simulink model "rpi_long_ctrl"  (R2022b)
settings: Solver=FixedStepAuto  StartTime=0.0  StopTime=15  RelTol=1e-3  EnableMultiTasking=on
values from neighbouring files (symbols this model uses):
  A = [1.06559801427  0.0478097134081  -0.0142426631232; 0.0478097134081  0.959164863261  -0.0359507847494; -0.0142426631232  -0.0359507847494  0.982079248423]    [matlab.mat]
  b = [2.14306210308 15.720848335 -0.863601368467]    [matlab.mat]
  D = 0    [matlab.mat]
  error_min = 0.04    [matlab.mat]
  I = 0    [matlab.mat]
  left_side = 0    [matlab.mat]
  N = 2    [matlab.mat]
  P = 1.25    [matlab.mat]
  pwm_k = 0.02    [matlab.mat]
  pwm_min = 0.27    [matlab.mat]
  pwm_min_ref = 0.25    [matlab.mat]
  target_scale = 0.75    [matlab.mat]
undefined symbols (not defined in the file or in its folder): ODR
libraries: raspberrypiBasiclib x6, simulink x2, raspberrypiIMUsensorslib x2, slpidlib x1, dspstat3 x1, dspsigops x1
settings Model: Creator=sjohnson  LastModifiedBy=sjohnson
settings SolverCC: PositivePriorityOrder=on
settings OptimizationCC: EnhancedBackFolding=on  PassReuseOutputArgsAs=Individual arguments  ZeroExternalMemoryAtStartup=off  ZeroInternalMemoryAtStartup=off  MaxStackSize=64  OptimizeBlockOrder=speed  DifferentSizesBufferReuse=on  OptimizationCustomize=off  EfficientTunableParamExpr=on
settings DebuggingCC: ParameterTunabilityLossMsg=error
settings HardwareCC: ProdBitPerPointer=32  ProdBitPerSizeT=32  ProdBitPerPtrDiffT=32  ProdLargestAtomicInteger=Long  ProdLargestAtomicFloat=Double  ProdWordSize=32  ProdLongLongMode=on  ProdHWDeviceType=ARM Compatible->ARM Cortex  UseEmbeddedCoderFeatures=off  UseSimulinkCoderFeatures=off
settings RTWCC: Description=Embedded Coder  SystemTargetFile=ert.tlc  HardwareBoard=Raspberry Pi  TLCOptions="-aInlineSetEventsForThisBaseRateFcn=TLC_FALSE -aSuppressMultiTaskScheduler=TLC_FALSE  -aRateBasedStepFcn=0"  TemplateMakefile=ert_default_tmf  Toolchain=GNU GCC Embedded Linux  BuildConfiguration=Faster Runs
settings CodeAppCC: ForceParamTrailComments=on  IgnoreCustomStorageClasses=off  OperatorAnnotations=on  SimulinkDataObjDesc=on  SFDataObjDesc=on  InsertBlockDesc=on
settings ERTTargetCC: SupportNonInlinedSFcns=on  SupportVariableSizeSignals=on  ExtModeTransport=2  ExtModeStaticAlloc=on  ExtModeMexFile=ext_xcp  ExtModeIntrfLevel=Level2 - Open

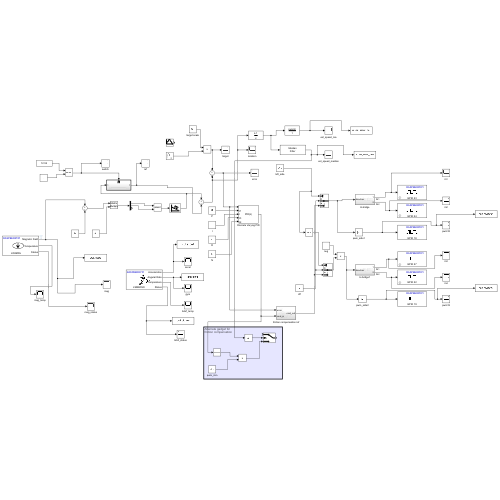
[thumbnail: Simulink's stored preview of the top-level diagram]
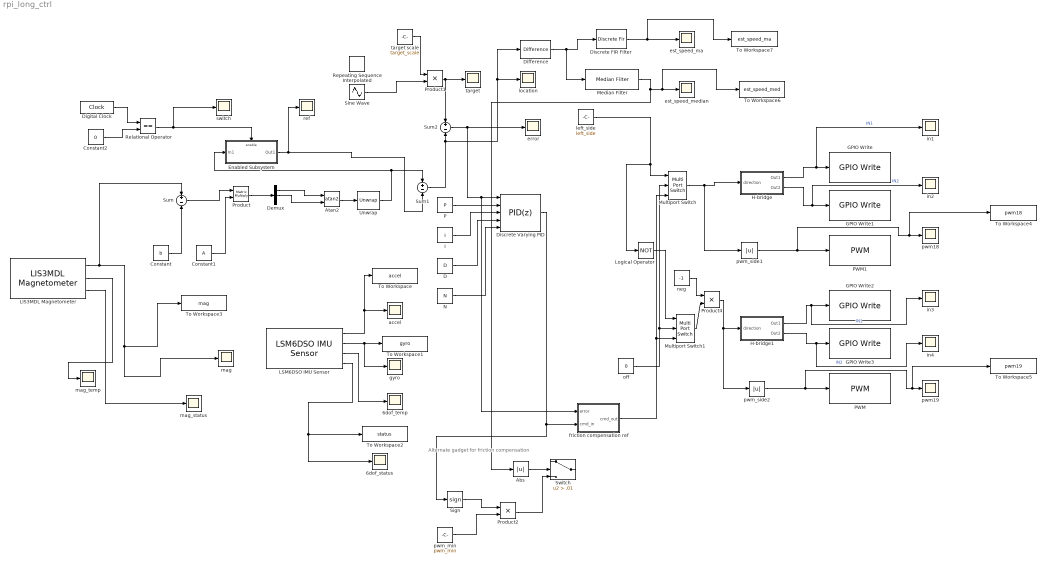
== system rpi_long_ctrl ==
  note: Alternate gadget for
      | friction compensation
  6dof_status : Scope
  6dof_temp : Scope
  Abs : Abs  SaturateOnIntegerOverflow=off
  Atan2 : Trigonometry  Operator=atan2
  Constant : Constant  Value=b
  Constant1 : Constant  Value=A
  Constant2 : Constant  Value=0
  D : Constant  Value=D
  Demux : Demux  Outputs=3
  Difference : simulink/Discrete/Difference  ICPrevInput=0  OutMin=[]  OutMax=[]  OutDataType=fixdt(1, 16)  OutScaling=2^-10  DoSatur=off
  Digital Clock : DigitalClock  SampleTime=0.04
  Discrete FIR Filter : DiscreteFir  Coefficients=[1 1 1 1 1]/5
  Discrete Varying PID : slpidlib/PID Controller  Controller=PID  Form=Parallel  TimeDomain=Discrete-time  UseExternalTs=off  SampleTime=-1  IntegratorMethod=Forward Euler  FilterMethod=Forward Euler  ControllerParametersSource=external  P=1  I=1  UseKiTs=off  D=0  N=100  UseFilter=on  TunerSelectOption=Transfer Function Based (PID Tuner App)  InitialConditionSource=internal  InitialConditionForIntegrator=0  InitialConditionForFilter=0  DifferentiatorICPrevScaledInput=0  ExternalReset=none  TrackingMode=off  Kt=1  LimitOutput=off  SatLimitsSource=internal  UpperSaturationLimit=inf  LowerSaturationLimit=-inf  LinearizeAsGain=on  AntiWindupMode=none  Kb=1  LimitIntegrator=off  UpperIntegratorSaturationLimit=inf  LowerIntegratorSaturationLimit=-inf  POutMin=[]  POutMax=[]  IOutMin=[]  IOutMax=[]  DOutMin=[]  DOutMax=[]  NOutMin=[]  NOutMax=[]  SumOutMin=[]  SumOutMax=[]  SaturationOutMin=[]  SaturationOutMax=[]  PParamMin=[]  PParamMax=[]  IParamMin=[]  IParamMax=[]  DParamMin=[]  DParamMax=[]  NParamMin=[]  NParamMax=[]  KbParamMin=[]  KbParamMax=[]  KtParamMin=[]  KtParamMax=[]  KbOutMin=[]  KbOutMax=[]  KtOutMin=[]  KtOutMax=[]  IntegratorOutMin=[]  IntegratorOutMax=[]  FilterOutMin=[]  FilterOutMax=[]  SumI1OutMin=[]  SumI1OutMax=[]  SumI2OutMin=[]  SumI2OutMax=[]  SumI3OutMin=[]  SumI3OutMax=[]  SumI4OutMin=[]  SumI4OutMax=[]  SumDOutMin=[]  SumDOutMax=[]  DifferentiatorOutMin=[]  DifferentiatorOutMax=[]  FilterDiffOutCoefMin=[]  FilterDiffOutCoefMax=[]  ReciprocalOutMin=[]  ReciprocalOutMax=[]  SumDenOutMin=[]  SumDenOutMax=[]  SumNumOutMin=[]  SumNumOutMax=[]  DivideOutMin=[]  DivideOutMax=[]  UdiffTsProdOutMin=[]  UdiffTsProdOutMax=[]  NTsProdOutMin=[]  NTsProdOutMax=[]  UintegralTsProdOutMin=[]  UintegralTsProdOutMax=[]  UngainTsProdOutMin=[]  UngainTsProdOutMax=[]  ClampingZeroOutDataTypeStr=Inherit: Inherit via back propagation  ClampingZeroOutMin=[]  ClampingZeroOutMax=[]  FilterDenConstantOutDataTypeStr=Inherit: Inherit via back propagation  FilterDenConstantOutMin=[]  FilterDenConstantOutMax=[]  PCopyOutDataTypeStr=Inherit: Inherit via back propagation  PCopyOutMin=[]  PCopyOutMax=[]  NCopyOutDataTypeStr=Inherit: Inherit via back propagation  NCopyOutMin=[]  NCopyOutMax=[]  IntegratorContinuousStateAttributes=''  IntegratorStateMustResolveToSignalObject=off  IntegratorRTWStateStorageClass=Auto  FilterContinuousStateAttributes=''  FilterStateMustResolveToSignalObject=off  FilterRTWStateStorageClass=Auto  ParallelPVariant=ExternalParameters  IdealPVariant=Disabled  IVariant=ExternalParameters  DVariant=ExternalParameters  IntegratorVariant=Discrete  SatVariant=Disabled  AWVariant=Passthrough  PCopyVariant=Disabled  TRVariant=Disabled  FdbkBlocksVariant=Forward  IdealPFdbkVariant=Disabled  SatFdbkVariant=Disabled  DerivativeFilterVariant=ForwardEulerFilter  NVariant=ExternalParameters  NCopyVariant=Disabled  FilterICVariant=InternalICsFilter  IntegratorICVariant=InternalICs  ExternalResetVariant=Disabled  TRSumVariant=Passthrough  SumFdbkVariant=Disabled  SumVariant=Sum_PID  TsampFilterVariant=InternalTs  TsampNgainVariant=Passthrough  TsampIntegralVariant=Passthrough  ExternalSaturationOutDataTypeStr=Inherit: Same as second input
      settings: LibrarySourceBlock=cstblocks/Linear Parameter Varying/Discrete Varying PID
  Enabled Subsystem : Subsystem  TreatAsAtomicUnit=on
  GPIO Write : raspberrypiBasiclib/GPIO Write  board=Pi 4 Model B  gpio=23  direction=Output  blockPlatform=Raspberry Pi
  GPIO Write1 : raspberrypiBasiclib/GPIO Write  board=Pi 4 Model B  gpio=24  direction=Output  blockPlatform=Raspberry Pi
  GPIO Write2 : raspberrypiBasiclib/GPIO Write  board=Pi 4 Model B  gpio=27  direction=Output  blockPlatform=Raspberry Pi
  GPIO Write3 : raspberrypiBasiclib/GPIO Write  board=Pi 4 Model B  gpio=22  direction=Output  blockPlatform=Raspberry Pi
  H-bridge : Subsystem
  H-bridge1 : Subsystem
  I : Constant  Value=I
  LIS3MDL Magnetometer : raspberrypiIMUsensorslib/LIS3MDL Magnetometer  I2CModule=1  I2CAddress=0x1E  IsActiveMagnetometer=on  IsActiveTemperature=on  IsStatus=on  SampleTime=-1  MagnetometerRange=+/- 400 uT  MagnetometerODR=40 Hz
  LSM6DSO IMU Sensor : raspberrypiIMUsensorslib/LSM6DSO IMU Sensor  I2CModule=1  I2CAddress=0x6B  IsActiveAcceleration=on  IsActiveAngularRate=on  IsActiveTemperature=on  IsActiveStatus=on  IsActiveTimeStamp=off  SampleTime=-1  QueueSizeFactor=3  AccelerometerRange=+/- 2g  AccelerometerODR=52 Hz  AccelSelectCompositeFilter=No filter  AccelLPF2BW=ODR/4  AccelHPFBW=ODR/4  GyroscopeRange=125 dps  GyroscopeODR=104 Hz  EnableGyroHPF=off  GyroHPFBW=0.016 Hz  EnableGyroLPF=off  GyroLPFBWMode=0
  Logical Operator : Logic  Operator=NOT  Inputs=1  AllPortsSameDT=off  OutDataTypeStr=boolean
  Median Filter : dspstat3/Median Filter  WindowLength=5  SimulateUsing=Interpreted execution
      settings: LibrarySourceBlock=|
      | dspfdesign/Median
      | Filter
  Multiport Switch : MultiPortSwitch  DataPortOrder=Zero-based contiguous  Inputs=2  zeroidx=on  SaturateOnIntegerOverflow=off  InputSameDT=off
  Multiport Switch1 : MultiPortSwitch  DataPortOrder=Zero-based contiguous  Inputs=2  zeroidx=on  SaturateOnIntegerOverflow=off  InputSameDT=off
  N : Constant  Value=N
  P : Constant  Value=P
  PWM : raspberrypiBasiclib/PWM  board=Pi 4 Model B  Pin_=19  Frequency=50  blockPlatform=Raspberry Pi
  PWM1 : raspberrypiBasiclib/PWM  board=Pi 4 Model B  Pin_=18  Frequency=50  blockPlatform=Raspberry Pi
  Product : Product  Multiplication=Matrix(*)
  Product1 : Product
  Product2 : Product
  Product4 : Product
  Relational Operator : RelationalOperator  Operator===  OutDataTypeStr=boolean  RndMeth=Simplest  InputSameDT=off
  Repeating Sequence Interpolated : simulink/Sources/Repeating Sequence Interpolated  OutValues=[0 pi/2 pi/2 pi pi pi/2 pi/2 0 0]  TimeValues=[0 1 2 3 4 5 6 7 8].'  LookUpMeth=Interpolation-Use End Values  tsamp=0.01  OutMin=[]  OutMax=[]  OutDataTypeStr=double  OutputDataTypeScalingMode=double  OutDataType=fixdt(0,8)  OutScaling=2^-10
  Sign : Signum
  Sine Wave : Sin  Amplitude=2*pi  Frequency=0.4  SampleTime=0.04
  Sum : Sum  Inputs=+-
  Sum1 : Sum  Inputs=+-
  Sum2 : Sum  Inputs=+-
  Switch : Switch  Criteria=u2 > Threshold  Threshold=.01  SaturateOnIntegerOverflow=off  InputSameDT=off
  To Workspace : ToWorkspace  VariableName=accel  SaveFormat=Structure With Time  SampleTime=-1
  To Workspace1 : ToWorkspace  VariableName=gyro  SaveFormat=Structure With Time  SampleTime=-1
  To Workspace2 : ToWorkspace  VariableName=status  SaveFormat=Structure With Time  SampleTime=-1
  To Workspace3 : ToWorkspace  VariableName=mag  SaveFormat=Structure With Time  SampleTime=-1
  To Workspace4 : ToWorkspace  VariableName=pwm18  SaveFormat=Structure With Time  SampleTime=-1
  To Workspace5 : ToWorkspace  VariableName=pwm19  SaveFormat=Structure With Time  SampleTime=-1
  To Workspace6 : ToWorkspace  VariableName=est_speed_med  SaveFormat=Structure With Time  SampleTime=-1
  To Workspace7 : ToWorkspace  VariableName=est_speed_ma  SaveFormat=Structure With Time  SampleTime=-1
  Unwrap : dspsigops/Unwrap  tol=pi  InputProcessing=Columns as channels (frame based)  running=off
  accel : Scope
  error : Scope
  est_speed_ma : Scope
  est_speed_median : Scope
  friction compensation ref : Subsystem
  gyro : Scope
  in{1..4} (4 alike) : Scope
  left_side : Constant  Value=left_side
  location : Scope
  mag : Scope
  mag_status : Scope
  mag_temp : Scope
  neg : Constant  Value=-1
  off : Constant  Value=0
  pwm18 : Scope
  pwm19 : Scope
  pwm_min : Constant  Value=pwm_min
  pwm_side1 : Abs  SaturateOnIntegerOverflow=off
  pwm_side2 : Abs  SaturateOnIntegerOverflow=off
  ref : Scope
  switch : Scope
  target : Scope
  target scale : Constant  Value=target_scale
  wires:
  Sine Wave/1 -> Product1/2
  LSM6DSO IMU Sensor/3 -> 6dof_temp/1
  LIS3MDL Magnetometer/3 -> mag_status/1
  LSM6DSO IMU Sensor/4 -> 6dof_status/1, To Workspace2/1
  LIS3MDL Magnetometer/1 -> Sum/1, To Workspace3/1, mag/1
  LSM6DSO IMU Sensor/1 -> accel/1, To Workspace/1
  LIS3MDL Magnetometer/2 -> mag_temp/1
  LSM6DSO IMU Sensor/2 -> gyro/1, To Workspace1/1
  Constant/1 -> Sum/2
  Sum/1 -> Product/1
  Constant1/1 -> Product/2
  Product/1 -> Demux/1
  Demux/1 -> Atan2/1
  Demux/2 -> Atan2/2
  Atan2/1 -> Unwrap/1
  Relational Operator/1 -> Enabled Subsystem/Enable, switch/1
  Digital Clock/1 -> Relational Operator/1
  Constant2/1 -> Relational Operator/2
  Enabled Subsystem/1(Out1) -> Sum1/2, ref/1
  Unwrap/1 -> Enabled Subsystem/1(In1), Sum1/1
  target scale/1 -> Product1/1
  Product1/1 -> target/1, Sum2/1
  off/1 -> Multiport Switch/2, Multiport Switch1/2
  Logical Operator/1 -> Multiport Switch1/1
  H-bridge1/2(Out2) -> in4/1, GPIO Write3/1  "IN2"
  left_side/1 -> Logical Operator/1, Multiport Switch/1
  pwm_side1/1 -> To Workspace4/1, pwm18/1, PWM1/1
  Product4/1 -> pwm_side2/1, H-bridge1/1(direction)
  pwm_side2/1 -> PWM/1, To Workspace5/1, pwm19/1
  H-bridge1/1(Out1) -> in3/1, GPIO Write2/1  "IN1"
  H-bridge/1(Out1) -> in1/1, GPIO Write/1  "IN1"
  Multiport Switch/1 -> pwm_side1/1, H-bridge/1(direction)
  H-bridge/2(Out2) -> in2/1, GPIO Write1/1  "IN2"
  Sum2/1 -> error/1, friction compensation ref/1(error), Discrete Varying PID/1
  P/1 -> Discrete Varying PID/2
  I/1 -> Discrete Varying PID/3
  D/1 -> Discrete Varying PID/4
  N/1 -> Discrete Varying PID/5
  neg/1 -> Product4/1
  Multiport Switch1/1 -> Product4/2
  Discrete Varying PID/1 -> Sign/1, friction compensation ref/2(cmd_in)
  Sum1/1 -> Difference/1, location/1, Sum2/2
  Difference/1 -> Median Filter/1, Discrete FIR Filter/1
  Discrete FIR Filter/1 -> To Workspace7/1, est_speed_ma/1
  Median Filter/1 -> Abs/1, To Workspace6/1, est_speed_median/1
  Abs/1 -> Switch/2
  Sign/1 -> Product2/1
  pwm_min/1 -> Product2/2
  Product2/1 -> Switch/3
  friction compensation ref/1(cmd_out) -> Multiport Switch1/3, Multiport Switch/3

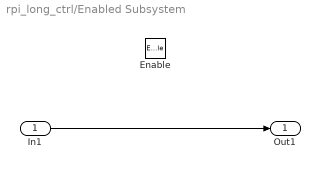
== system rpi_long_ctrl/Enabled Subsystem ==
  In1 : Inport
  Enable : EnablePort
  Out1 : Outport
  wires:
  In1/1 -> Out1/1

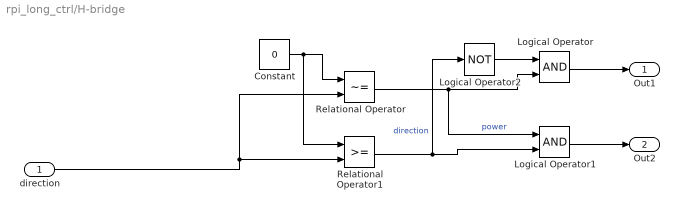
== system rpi_long_ctrl/H-bridge ==
  direction : Inport
  Constant : Constant  Value=0
  Logical Operator : Logic  AllPortsSameDT=off  OutDataTypeStr=boolean
  Logical Operator1 : Logic  AllPortsSameDT=off  OutDataTypeStr=boolean
  Logical Operator2 : Logic  Operator=NOT  Inputs=1  AllPortsSameDT=off  OutDataTypeStr=boolean
  Relational Operator : RelationalOperator  Operator=~=  OutDataTypeStr=boolean  RndMeth=Simplest  InputSameDT=off
  Relational Operator1 : RelationalOperator  OutDataTypeStr=boolean  RndMeth=Simplest  InputSameDT=off
  Out1 : Outport
  Out2 : Outport  Port=2
  wires:
  Logical Operator/1 -> Out1/1
  Relational Operator1/1 -> Logical Operator2/1, Logical Operator1/2  "direction"
  Logical Operator1/1 -> Out2/1
  Logical Operator2/1 -> Logical Operator/1
  direction/1 -> Relational Operator/2, Relational Operator1/2
  Constant/1 -> Relational Operator1/1, Relational Operator/1
  Relational Operator/1 -> Logical Operator1/1, Logical Operator/2  "power"

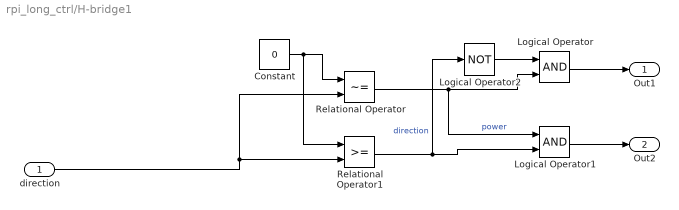
== system rpi_long_ctrl/H-bridge1 ==
  direction : Inport
  Constant : Constant  Value=0
  Logical Operator : Logic  AllPortsSameDT=off  OutDataTypeStr=boolean
  Logical Operator1 : Logic  AllPortsSameDT=off  OutDataTypeStr=boolean
  Logical Operator2 : Logic  Operator=NOT  Inputs=1  AllPortsSameDT=off  OutDataTypeStr=boolean
  Relational Operator : RelationalOperator  Operator=~=  OutDataTypeStr=boolean  RndMeth=Simplest  InputSameDT=off
  Relational Operator1 : RelationalOperator  OutDataTypeStr=boolean  RndMeth=Simplest  InputSameDT=off
  Out1 : Outport
  Out2 : Outport  Port=2
  wires:
  Logical Operator/1 -> Out1/1
  Relational Operator1/1 -> Logical Operator2/1, Logical Operator1/2  "direction"
  Logical Operator1/1 -> Out2/1
  Logical Operator2/1 -> Logical Operator/1
  direction/1 -> Relational Operator/2, Relational Operator1/2
  Constant/1 -> Relational Operator1/1, Relational Operator/1
  Relational Operator/1 -> Logical Operator1/1, Logical Operator/2  "power"

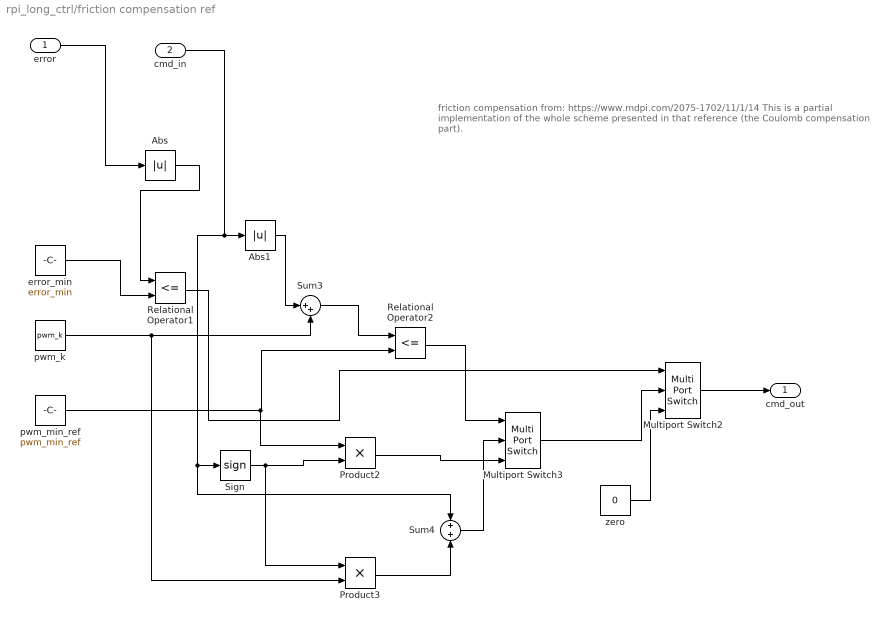
== system rpi_long_ctrl/friction compensation ref ==
  note: friction compensation from:
      | https://www.mdpi.com/2075-1702/11/1/14
      | This is a partial implementation of the whole scheme presented in that reference (the Coulomb compensation part).
  error : Inport
  cmd_in : Inport  Port=2
  Abs : Abs  SaturateOnIntegerOverflow=off
  Abs1 : Abs  SaturateOnIntegerOverflow=off
  Multiport Switch2 : MultiPortSwitch  DataPortOrder=Zero-based contiguous  Inputs=2  zeroidx=on  SaturateOnIntegerOverflow=off  InputSameDT=off
  Multiport Switch3 : MultiPortSwitch  DataPortOrder=Zero-based contiguous  Inputs=2  zeroidx=on  SaturateOnIntegerOverflow=off  InputSameDT=off
  Product2 : Product
  Product3 : Product
  Relational Operator1 : RelationalOperator  Operator=<=  OutDataTypeStr=boolean  RndMeth=Simplest  InputSameDT=off
  Relational Operator2 : RelationalOperator  Operator=<=  OutDataTypeStr=boolean  RndMeth=Simplest  InputSameDT=off
  Sign : Signum
  Sum3 : Sum  Inputs=|++
  Sum4 : Sum
  error_min : Constant  Value=error_min
  pwm_k : Constant  Value=pwm_k
  pwm_min_ref : Constant  Value=pwm_min_ref
  zero : Constant  Value=0
  cmd_out : Outport
  wires:
  cmd_in/1 -> Sum4/1, Sign/1, Abs1/1
  Relational Operator1/1 -> Multiport Switch2/1
  zero/1 -> Multiport Switch2/3
  Sum3/1 -> Relational Operator2/1
  Product2/1 -> Multiport Switch3/3
  Sign/1 -> Product3/1, Product2/2
  Product3/1 -> Sum4/2
  Relational Operator2/1 -> Multiport Switch3/1
  Multiport Switch2/1 -> cmd_out/1
  error/1 -> Abs/1
  pwm_min_ref/1 -> Product2/1, Relational Operator2/2
  error_min/1 -> Relational Operator1/2
  pwm_k/1 -> Product3/2, Sum3/2
  Abs/1 -> Relational Operator1/1
  Abs1/1 -> Sum3/1
  Multiport Switch3/1 -> Multiport Switch2/2
  Sum4/1 -> Multiport Switch3/2
